simulink library "generator_lib"  (Simulink 7.8)
settings: Solver=ode45  StartTime=0.0  StopTime=10.0  RelTol=1e-3
undefined symbols (not defined in the file): dfilt, DiscIntNeverNeededParam, fdesignblkfcn, gcbh, ph, Ts
libraries: simulink x91, rtio_opalrt_common x84, powerlib x51, simulink_extras x21, discretizing x14, rteventslib x14, dsparch4 x14, powerlib_extras x4
(part 10 of 10)

== system generator_lib/Generator_09112015/GenSet_1MVA_09082015/900kW Generator with  Primary Controllers/Diesel Engine Speed & Voltage Control fast/Excitation/Exciter  1 / (te.s + ke)/1st order Lowpass ==
  In : Inport
  Discrete State-Space : DiscreteStateSpace  A=Ad  B=Bd  C=Cd  D=Dd  X0=x0d  SampleTime=Ts
  Out : Outport  InitialOutput=0
  wires:
  In/1 -> Discrete State-Space/1
  Discrete State-Space/1 -> Out/1

== system generator_lib/Generator_09112015/GenSet_1MVA_09082015/900kW Generator with  Primary Controllers/Diesel Engine Speed & Voltage Control fast/Excitation/Main Regulator ka / (ta.s +1)/1st order Lowpass ==
  In : Inport
  Discrete State-Space : DiscreteStateSpace  A=Ad  B=Bd  C=Cd  D=Dd  X0=x0d  SampleTime=Ts
  Out : Outport  InitialOutput=0
  wires:
  In/1 -> Discrete State-Space/1
  Discrete State-Space/1 -> Out/1

== system generator_lib/Generator_09112015/GenSet_4MVA_copy1mva/4MVA Generator with  Primary Controllers/Diesel Engine Speed & Voltage Control fast/Excitation/Damping kf.s / (tf.s +1)/1st-Order Discrete Filter ==
  In : Inport
  Discrete State-Space : DiscreteStateSpace  A=Ad  B=Bd  C=Cd  D=Dd  X0=x0d  SampleTime=Ts
  Out : Outport  InitialOutput=0
  wires:
  In/1 -> Discrete State-Space/1
  Discrete State-Space/1 -> Out/1

== system generator_lib/Generator_09112015/GenSet_4MVA_copy1mva/4MVA Generator with  Primary Controllers/Diesel Engine Speed & Voltage Control fast/Excitation/Exciter  1 / (te.s + ke)/1st order Lowpass ==
  In : Inport
  Discrete State-Space : DiscreteStateSpace  A=Ad  B=Bd  C=Cd  D=Dd  X0=x0d  SampleTime=Ts
  Out : Outport  InitialOutput=0
  wires:
  In/1 -> Discrete State-Space/1
  Discrete State-Space/1 -> Out/1

== system generator_lib/Generator_09112015/GenSet_4MVA_copy1mva/4MVA Generator with  Primary Controllers/Diesel Engine Speed & Voltage Control fast/Excitation/Main Regulator ka / (ta.s +1)/1st order Lowpass ==
  In : Inport
  Discrete State-Space : DiscreteStateSpace  A=Ad  B=Bd  C=Cd  D=Dd  X0=x0d  SampleTime=Ts
  Out : Outport  InitialOutput=0
  wires:
  In/1 -> Discrete State-Space/1
  Discrete State-Space/1 -> Out/1

== system generator_lib/Generator_09142015/GenSet_1MVA_09082015/900kW Generator with  Primary Controllers/Diesel Engine Speed & Voltage Control fast/Excitation/Damping kf.s / (tf.s +1)/1st-Order Discrete Filter ==
  In : Inport
  Discrete State-Space : DiscreteStateSpace  A=Ad  B=Bd  C=Cd  D=Dd  X0=x0d  SampleTime=Ts
  Out : Outport  InitialOutput=0
  wires:
  Discrete State-Space/1 -> Out/1
  In/1 -> Discrete State-Space/1

== system generator_lib/Generator_09142015/GenSet_1MVA_09082015/900kW Generator with  Primary Controllers/Diesel Engine Speed & Voltage Control fast/Excitation/Exciter  1 / (te.s + ke)/1st order Lowpass ==
  In : Inport
  Discrete State-Space : DiscreteStateSpace  A=Ad  B=Bd  C=Cd  D=Dd  X0=x0d  SampleTime=Ts
  Out : Outport  InitialOutput=0
  wires:
  Discrete State-Space/1 -> Out/1
  In/1 -> Discrete State-Space/1

== system generator_lib/Generator_09142015/GenSet_1MVA_09082015/900kW Generator with  Primary Controllers/Diesel Engine Speed & Voltage Control fast/Excitation/Main Regulator ka / (ta.s +1)/1st order Lowpass ==
  In : Inport
  Discrete State-Space : DiscreteStateSpace  A=Ad  B=Bd  C=Cd  D=Dd  X0=x0d  SampleTime=Ts
  Out : Outport  InitialOutput=0
  wires:
  Discrete State-Space/1 -> Out/1
  In/1 -> Discrete State-Space/1

== system generator_lib/Generator_09142015/GenSet_4MVA_09142015/4MVA Generator with  Primary Controllers/Diesel Engine Speed & Voltage Control fast/Excitation/Damping kf.s / (tf.s +1)/1st-Order Discrete Filter ==
  In : Inport
  Discrete State-Space : DiscreteStateSpace  A=Ad  B=Bd  C=Cd  D=Dd  X0=x0d  SampleTime=Ts
  Out : Outport  InitialOutput=0
  wires:
  Discrete State-Space/1 -> Out/1
  In/1 -> Discrete State-Space/1

== system generator_lib/Generator_09142015/GenSet_4MVA_09142015/4MVA Generator with  Primary Controllers/Diesel Engine Speed & Voltage Control fast/Excitation/Exciter  1 / (te.s + ke)/1st order Lowpass ==
  In : Inport
  Discrete State-Space : DiscreteStateSpace  A=Ad  B=Bd  C=Cd  D=Dd  X0=x0d  SampleTime=Ts
  Out : Outport  InitialOutput=0
  wires:
  Discrete State-Space/1 -> Out/1
  In/1 -> Discrete State-Space/1

== system generator_lib/Generator_09142015/GenSet_4MVA_09142015/4MVA Generator with  Primary Controllers/Diesel Engine Speed & Voltage Control fast/Excitation/Main Regulator ka / (ta.s +1)/1st order Lowpass ==
  In : Inport
  Discrete State-Space : DiscreteStateSpace  A=Ad  B=Bd  C=Cd  D=Dd  X0=x0d  SampleTime=Ts
  Out : Outport  InitialOutput=0
  wires:
  Discrete State-Space/1 -> Out/1
  In/1 -> Discrete State-Space/1

== system generator_lib/Generator_09152015/GenSet_1MVA_09082015/900kW Generator with  Primary Controllers/Diesel Engine Speed & Voltage Control fast/Excitation/Damping kf.s / (tf.s +1)/1st-Order Discrete Filter ==
  In : Inport
  Discrete State-Space : DiscreteStateSpace  A=Ad  B=Bd  C=Cd  D=Dd  X0=x0d  SampleTime=Ts
  Out : Outport  InitialOutput=0
  wires:
  Discrete State-Space/1 -> Out/1
  In/1 -> Discrete State-Space/1

== system generator_lib/Generator_09152015/GenSet_1MVA_09082015/900kW Generator with  Primary Controllers/Diesel Engine Speed & Voltage Control fast/Excitation/Exciter  1 / (te.s + ke)/1st order Lowpass ==
  In : Inport
  Discrete State-Space : DiscreteStateSpace  A=Ad  B=Bd  C=Cd  D=Dd  X0=x0d  SampleTime=Ts
  Out : Outport  InitialOutput=0
  wires:
  Discrete State-Space/1 -> Out/1
  In/1 -> Discrete State-Space/1

== system generator_lib/Generator_09152015/GenSet_1MVA_09082015/900kW Generator with  Primary Controllers/Diesel Engine Speed & Voltage Control fast/Excitation/Main Regulator ka / (ta.s +1)/1st order Lowpass ==
  In : Inport
  Discrete State-Space : DiscreteStateSpace  A=Ad  B=Bd  C=Cd  D=Dd  X0=x0d  SampleTime=Ts
  Out : Outport  InitialOutput=0
  wires:
  Discrete State-Space/1 -> Out/1
  In/1 -> Discrete State-Space/1

== system generator_lib/Generator_09152015/GenSet_4MVA_09142015/4MVA Generator with  Primary Controllers/Diesel Engine Speed & Voltage Control fast/Excitation/Damping kf.s / (tf.s +1)/1st-Order Discrete Filter ==
  In : Inport
  Discrete State-Space : DiscreteStateSpace  A=Ad  B=Bd  C=Cd  D=Dd  X0=x0d  SampleTime=Ts
  Out : Outport  InitialOutput=0
  wires:
  Discrete State-Space/1 -> Out/1
  In/1 -> Discrete State-Space/1

== system generator_lib/Generator_09152015/GenSet_4MVA_09142015/4MVA Generator with  Primary Controllers/Diesel Engine Speed & Voltage Control fast/Excitation/Exciter  1 / (te.s + ke)/1st order Lowpass ==
  In : Inport
  Discrete State-Space : DiscreteStateSpace  A=Ad  B=Bd  C=Cd  D=Dd  X0=x0d  SampleTime=Ts
  Out : Outport  InitialOutput=0
  wires:
  Discrete State-Space/1 -> Out/1
  In/1 -> Discrete State-Space/1

== system generator_lib/Generator_09152015/GenSet_4MVA_09142015/4MVA Generator with  Primary Controllers/Diesel Engine Speed & Voltage Control fast/Excitation/Main Regulator ka / (ta.s +1)/1st order Lowpass ==
  In : Inport
  Discrete State-Space : DiscreteStateSpace  A=Ad  B=Bd  C=Cd  D=Dd  X0=x0d  SampleTime=Ts
  Out : Outport  InitialOutput=0
  wires:
  Discrete State-Space/1 -> Out/1
  In/1 -> Discrete State-Space/1
